simulink library "cooperative"  (Simulink 7.4)
settings: Solver=ode45  SolverMode=SingleTasking  StartTime=0.0  StopTime=10.0  RelTol=1e-3
undefined symbols (not defined in the file): ATRFunctions, g_AssignmentAlgorithm, g_CommandTurnRadius, g_CoordinationDelayDen, g_DefaultWaypointAltitude, g_EntityTypes, g_MaxNumberTargets, g_MaxNumberVehicles, g_MaxReassignmentDeltaTime, g_ObjectMessageIDs, g_OptionSaveDataAVDS, g_SampleTime, g_SensorRollLimitDeg, g_TargetStates, g_Tasks, g_TruthMemory, g_TypeAssignment, g_VehicleInputFiles, g_VehicleMemory, g_VehicleTypes, g_WaypointDefinitions, g_WaypointTypes
libraries: cooperative x23
(part 2 of 3)

== system cooperative/UAV1/SendMessages/SendATRTime ==
  VehicleID : Inport
  CommBusLocal : Inport  Port=2
  Bus Selector1 : BusSelector  OutputSignals=EFS(com).SensorManager(com).ATR Single.ATR Time
  CreateWaypointIndex : DataStoreMemory  DataStoreName=ATRTime
  Enabled Subsystem : Subsystem  TreatAsAtomicUnit=on
  Mux2 : Mux
  ReadWaypointIndex : DataStoreRead  DataStoreName=ATRTime  SampleTime=g_SampleTime
  Relational Operator : RelationalOperator  Operator=~=  InputSameDT=on
  SendATRTime : cooperative/SendMessage  ReuseMatrix=growing  MessageTypeStr=ATRTime
  Terminator : Terminator
  VehicleOffset : Constant  Value=g_ObjectMessageIDs.AllVehiclesTypeShifted + 1
  wires:
  Bus Selector1/1 -> Enabled Subsystem/1(ATRTime), Relational Operator/2, Mux2/3  "<ATR Time>"
  Enabled Subsystem/1(TimeStamp) -> Mux2/2  "TimeStamp"
  Mux2/1 -> SendATRTime/1
  Relational Operator/1 -> Enabled Subsystem/Enable
  ReadWaypointIndex/1 -> Relational Operator/1
  VehicleID/1 -> Mux2/1
  CommBusLocal/1 -> Bus Selector1/1
  VehicleOffset/1 -> Mux2/4
  SendATRTime/1 -> Terminator/1

== system cooperative/UAV1/SendMessages/SendAuctionData ==
  VehicleID : Inport
  CommBusLocal : Inport  Port=2
  Bus Selector1 : BusSelector  OutputSignals=EFS(com).CooperationManager(com).AuctionData.MessageNumber,EFS(com).CooperationManager(com).AuctionData.ReplanRound,EFS(com).CooperationManager(com).AuctionData.BidTarget,EFS(com).CooperationManager(com).AuctionData.BidPrice,EFS(com).CooperationManager(com).AuctionData.BidTargetETA,EFS(com).CooperationManager(com).AuctionData.AssignedTarget,EFS(com).CooperationManager(com).AuctionData.AssignedPrice,EFS(com).CooperationManager(com).AuctionData.AssignedTargetETA
  Data Store Memory : DataStoreMemory  DataStoreName=LastMessageNumber
  Data Store Read : DataStoreRead  DataStoreName=LastMessageNumber  SampleTime=g_SampleTime
  Enabled Subsystem : Subsystem  Priority=1  TreatAsAtomicUnit=on
  Mux2 : Mux  Inputs=11
  Relational Operator : RelationalOperator  Operator=~=  InputSameDT=on
  "SendAuctionData " : cooperative/SendMessage  Priority=2  ReuseMatrix=growing  MessageTypeStr=AuctionData
  Sum : Sum  Inputs=+  SaturateOnIntegerOverflow=on  InputSameDT=on  OutDataTypeStr=Inherit: Same as first input
  Terminator : Terminator
  VehicleOffset : Constant  Value=g_ObjectMessageIDs.AllVehiclesTypeShifted + 1
  wires:
  Bus Selector1/1 -> Enabled Subsystem/1(MessageNumber), Relational Operator/2  "<MessageNumber>"
  Bus Selector1/2 -> Mux2/4  "<ReplanRound>"
  Bus Selector1/3 -> Mux2/5  "<BidTarget>"
  Bus Selector1/4 -> Mux2/6  "<BidPrice>"
  Bus Selector1/5 -> Mux2/7  "<BidTargetETA>"
  Bus Selector1/6 -> Mux2/8  "<AssignedTarget>"
  Bus Selector1/7 -> Mux2/9  "<AssignedPrice>"
  Bus Selector1/8 -> Mux2/10  "<AssignedTargetETA>"
  Sum/1 -> Enabled Subsystem/Enable
  Relational Operator/1 -> Sum/1
  Data Store Read/1 -> Relational Operator/1
  Enabled Subsystem/1(TimeStamp) -> Mux2/3, Mux2/2  "TimeStamp"
  Mux2/1 -> "SendAuctionData "/1
  VehicleID/1 -> Mux2/1
  CommBusLocal/1 -> Bus Selector1/1
  VehicleOffset/1 -> Mux2/11
  "SendAuctionData "/1 -> Terminator/1

== system cooperative/UAV1/SendMessages/SendChangedStatus ==
  VehicleID : Inport
  CommBusLocal : Inport  Port=2
  Bus Selector1 : BusSelector  OutputSignals=EFS(com).TargetManager(com).Target Status.ChangedStatus
  Enabled Subsystem : Subsystem  TreatAsAtomicUnit=on
  Mux2 : Mux
  "SendChangedStatus " : cooperative/SendMessage  ReuseMatrix=growing  MessageTypeStr=ChangedStatus
  Terminator : Terminator
  VehicleOffset : Constant  Value=g_ObjectMessageIDs.AllVehiclesTypeShifted + 1
  wires:
  Bus Selector1/1 -> Enabled Subsystem/Enable, Mux2/3  "<ChangedStatus>"
  Enabled Subsystem/1(TimeStamp) -> Mux2/2  "TimeStamp"
  Mux2/1 -> "SendChangedStatus "/1
  VehicleID/1 -> Mux2/1
  CommBusLocal/1 -> Bus Selector1/1
  VehicleOffset/1 -> Mux2/4
  "SendChangedStatus "/1 -> Terminator/1

== system cooperative/UAV1/SendMessages/SendETAsCostsReturnToSearch ==
  VehicleID : Inport
  CommBusLocal : Inport  Port=2
  Bus Selector2 : BusSelector  OutputSignals=EFS(com).RouteManager(com).Replan ETAs and Costs.ReplanTime,EFS(com).RouteManager(com).Replan ETAs and Costs  OutputAsBus=on
  Mux : Mux  Inputs=3
  SendETAsCostsReturnToSearch : cooperative/SendMessage  ReuseMatrix=growing  MessageTypeStr=ETACostToSearch
  Terminator : Terminator
  VehicleOffset : Constant  Value=g_ObjectMessageIDs.AllVehiclesTypeShifted + 1
  wires:
  CommBusLocal/1 -> Bus Selector2/1
  VehicleID/1 -> Mux/1
  Mux/1 -> SendETAsCostsReturnToSearch/1
  Bus Selector2/1 -> Mux/2
  VehicleOffset/1 -> Mux/3
  SendETAsCostsReturnToSearch/1 -> Terminator/1

== system cooperative/UAV1/SendMessages/SendPositionFlag ==
  VehicleID : Inport
  CommBusLocal : Inport  Port=2
  CommBus : Inport  Port=3
  Bus Selector1 : BusSelector  OutputSignals=EFS(com).TargetManager(com).Target Status.NewTarget,EFS(com).RouteManager(com).NewPlans  OutputAsBus=on
  Bus Selector2 : BusSelector  OutputSignals=TimeTriggerReplan  OutputAsBus=on
  CreateWaypointIndex : DataStoreMemory  DataStoreName=PositionFlag  InitialValue=[0 0 0]
  Enabled Subsystem : Subsystem  TreatAsAtomicUnit=on
  Logical Operator1 : Logic  Operator=OR  Inputs=1
  Mux : Mux  Inputs=2
  Mux2 : Mux
  ReadWaypointIndex : DataStoreRead  DataStoreName=PositionFlag  SampleTime=g_SampleTime
  Relational Operator : RelationalOperator  Operator=~=  InputSameDT=on
  SendATRTime : cooperative/SendMessage  ReuseMatrix=growing  MessageTypeStr=SendPositionsFlag
  Terminator : Terminator
  VehicleOffset : Constant  Value=g_ObjectMessageIDs.AllVehiclesTypeShifted + 1
  wires:
  Mux/1 -> Enabled Subsystem/1(PositionFlag), Relational Operator/2
  Bus Selector1/1 -> Mux/1
  Bus Selector2/1 -> Mux/2
  CommBus/1 -> Bus Selector2/1
  Logical Operator1/1 -> Mux2/3, Enabled Subsystem/Enable
  Relational Operator/1 -> Logical Operator1/1
  CommBusLocal/1 -> Bus Selector1/1
  VehicleID/1 -> Mux2/1
  ReadWaypointIndex/1 -> Relational Operator/1
  Mux2/1 -> SendATRTime/1
  Enabled Subsystem/1(TimeStamp) -> Mux2/2  "TimeStamp"
  VehicleOffset/1 -> Mux2/4
  SendATRTime/1 -> Terminator/1

== system cooperative/UAV1/SendMessages/SendPositionID ==
  note: NOTE: Since the received messages are not reset to zero after they are handled, it was necessary to reset the PositionsFlag signal here.
      | The issue of resetting the message values to zero may be moved into the S-Function.
  VehicleID : Inport
  CommBusLocal : Inport  Port=2
  CommBus : Inport  Port=3
  Bus Selector1 : BusSelector  OutputSignals=Dynamics(com).AC Dynamics.Position_x,Dynamics(com).AC Dynamics.Position_y,Dynamics(com).AC Dynamics.Psi  OutputAsBus=on
  Bus Selector2 : BusSelector  OutputSignals=TimePositionsFlag  OutputAsBus=on
  Data Store Memory : DataStoreMemory  DataStoreName=PositionsSendFlagTime
  Data Store Read : DataStoreRead  DataStoreName=PositionsSendFlagTime  SampleTime=g_SampleTime
  Enabled Subsystem : Subsystem  TreatAsAtomicUnit=on
  Mux2 : Mux  Inputs=5
  Relational Operator : RelationalOperator  Operator=~=  InputSameDT=on
  "SendPositionID " : cooperative/SendMessage  ReuseMatrix=growing  MessageTypeStr=PositionID
  Terminator : Terminator
  VehicleOffset : Constant  Value=g_ObjectMessageIDs.AllVehiclesTypeShifted + 1
  wires:
  Relational Operator/1 -> Enabled Subsystem/Enable
  Data Store Read/1 -> Relational Operator/1
  Bus Selector2/1 -> Relational Operator/2, Enabled Subsystem/1(PositionSendFlag Time)
  CommBus/1 -> Bus Selector2/1
  CommBusLocal/1 -> Bus Selector1/1
  VehicleID/1 -> Mux2/3, Mux2/1
  Mux2/1 -> "SendPositionID "/1
  Enabled Subsystem/1(TimeStamp) -> Mux2/2  "TimeStamp"
  Bus Selector1/1 -> Mux2/4
  VehicleOffset/1 -> Mux2/5
  "SendPositionID "/1 -> Terminator/1

== system cooperative/UAV1/SendMessages/SendTargetAttacked ==
  VehicleID : Inport
  CommBusLocal : Inport  Port=2
  Bus Selector1 : BusSelector  OutputSignals=EFS(com).RouteManager(com).TaskStatus.Target Attacked
  CreateWaypointIndex : DataStoreMemory  DataStoreName=TargetAttacked
  Enabled Subsystem : Subsystem  TreatAsAtomicUnit=on
  Mux2 : Mux
  ReadWaypointIndex : DataStoreRead  DataStoreName=TargetAttacked  SampleTime=g_SampleTime
  Relational Operator : RelationalOperator  Operator=~=  InputSameDT=on
  "SendTargetAttacked " : cooperative/SendMessage  ReuseMatrix=growing  MessageTypeStr=TargetAttacked
  Terminator : Terminator
  VehicleOffset : Constant  Value=g_ObjectMessageIDs.AllVehiclesTypeShifted + 1
  wires:
  CommBusLocal/1 -> Bus Selector1/1
  VehicleID/1 -> Mux2/1
  ReadWaypointIndex/1 -> Relational Operator/1
  Relational Operator/1 -> Enabled Subsystem/Enable
  Mux2/1 -> "SendTargetAttacked "/1
  Enabled Subsystem/1(TimeStamp) -> Mux2/2  "TimeStamp"
  Bus Selector1/1 -> Mux2/3, Relational Operator/2, Enabled Subsystem/1("TargetAttacked ")  "<Target Attacked>"
  VehicleOffset/1 -> Mux2/4
  "SendTargetAttacked "/1 -> Terminator/1

== system cooperative/UAV1/SendMessages/SendTargetStatus ==
  VehicleID : Inport
  CommBusLocal : Inport  Port=2
  Bus Selector1 : BusSelector  OutputSignals=EFS(com).TargetManager(com).TargetStatusNoDelay.TargetStatus
  Bus Selector2 : BusSelector  OutputSignals=EFS(com).TargetManager(com).TargetStatusNoDelay.ChangedStatus
  Enabled Subsystem : Subsystem  Priority=1  TreatAsAtomicUnit=on
  Mux2 : Mux
  "SendTargetStatus " : cooperative/SendMessage  Priority=2  ReuseMatrix=growing  MessageTypeStr=TargetStatus
  Terminator : Terminator
  VehicleOffset : Constant  Value=g_ObjectMessageIDs.AllVehiclesTypeShifted + 1
  wires:
  Bus Selector2/1 -> Enabled Subsystem/Enable  "<ChangedStatus>"
  Bus Selector1/1 -> Mux2/3  "<TargetStatus>"
  Enabled Subsystem/1(TimeStamp) -> Mux2/2  "TimeStamp"
  Mux2/1 -> "SendTargetStatus "/1
  VehicleID/1 -> Mux2/1
  CommBusLocal/1 -> Bus Selector2/1, Bus Selector1/1
  VehicleOffset/1 -> Mux2/4
  "SendTargetStatus "/1 -> Terminator/1

== system cooperative/UAV1/SendMessages/SendTaskBenefits ==
  VehicleID : Inport
  CommBusLocal : Inport  Port=2
  Bus Selector1 : BusSelector  OutputSignals=EFS(com).CooperationManager(com).Algorithm Data.ReplanRound,EFS(com).CooperationManager(com).Algorithm Data.TargetStates,EFS(com).CooperationManager(com).Algorithm Data.TaskBenefits,EFS(com).CooperationManager(com).Algorithm Data.TimeToComplete,EFS(com).CooperationManager(com).Algorithm Data.SearchBenefit
  Data Store Memory : DataStoreMemory  DataStoreName=LastReplanRound  InitialValue=[0;0]
  Data Store Read : DataStoreRead  DataStoreName=LastReplanRound  SampleTime=g_SampleTime
  Enabled Subsystem : Subsystem  Priority=1  TreatAsAtomicUnit=on
  Mux2 : Mux  Inputs=8
  Relational Operator : RelationalOperator  Operator=~=  InputSameDT=on
  "SendTaskBenefits " : cooperative/SendMessage  Priority=2  ReuseMatrix=growing  MessageTypeStr=TaskBenefits
  Sum : Sum  Inputs=+  SaturateOnIntegerOverflow=on  InputSameDT=on  OutDataTypeStr=Inherit: Same as first input
  Terminator : Terminator
  VehicleOffset : Constant  Value=g_ObjectMessageIDs.AllVehiclesTypeShifted + 1
  wires:
  Bus Selector1/5 -> Mux2/7  "<SearchBenefit>"
  Bus Selector1/4 -> Mux2/6  "<TimeToComplete>"
  Bus Selector1/3 -> Mux2/5  "<TaskBenefits>"
  Sum/1 -> Enabled Subsystem/Enable
  Relational Operator/1 -> Sum/1
  Data Store Read/1 -> Relational Operator/1
  Bus Selector1/2 -> Mux2/4  "<TargetStates>"
  Bus Selector1/1 -> Enabled Subsystem/1(ReplanRound), Relational Operator/2, Mux2/3  "<ReplanRound>"
  Enabled Subsystem/1(TimeStamp) -> Mux2/2  "TimeStamp"
  Mux2/1 -> "SendTaskBenefits "/1
  VehicleID/1 -> Mux2/1
  CommBusLocal/1 -> Bus Selector1/1
  VehicleOffset/1 -> Mux2/8
  "SendTaskBenefits "/1 -> Terminator/1

== system cooperative/UAV1/SendMessages/SendTriggerReplan ==
  VehicleID : Inport
  CommBusLocal : Inport  Port=2
  Bus Selector1 : BusSelector  OutputSignals=EFS(com).RouteManager(com).TaskStatus.TriggerReplan  OutputAsBus=on
  Enabled Subsystem : Subsystem  TreatAsAtomicUnit=on
  Mux1 : Mux
  SendTriggerReplan : cooperative/SendMessage  ReuseMatrix=growing  MessageTypeStr=TriggerReplan
  Terminator : Terminator
  VehicleOffset : Constant  Value=g_ObjectMessageIDs.AllVehiclesTypeShifted + 1
  wires:
  Enabled Subsystem/1(TimeStamp) -> Mux1/2  "TriggerReplanTriggered"
  Bus Selector1/1 -> Enabled Subsystem/Enable, Mux1/3
  CommBusLocal/1 -> Bus Selector1/1
  VehicleID/1 -> Mux1/1
  Mux1/1 -> SendTriggerReplan/1
  VehicleOffset/1 -> Mux1/4
  SendTriggerReplan/1 -> Terminator/1

== system cooperative/UAV1/SendMessages/SendWaypointNumber ==
  VehicleID : Inport
  CommBusLocal : Inport  Port=2
  Bus Selector1 : BusSelector  OutputSignals=Dynamics(com).TacticalManuevering.WayPointNumber
  CreateWaypointIndex : DataStoreMemory  DataStoreName=WaypoinNumber  InitialValue=1
  Enabled Subsystem : Subsystem  TreatAsAtomicUnit=on
  Mux2 : Mux
  ReadWaypointIndex : DataStoreRead  DataStoreName=WaypoinNumber  SampleTime=g_SampleTime
  Relational Operator : RelationalOperator  Operator=~=  InputSameDT=on
  SendWaypointIndex : cooperative/SendMessage  ReuseMatrix=growing  MessageTypeStr=WaypointIndex
  Terminator : Terminator
  VehicleOffset : Constant  Value=g_ObjectMessageIDs.AllVehiclesTypeShifted + 1
  wires:
  CommBusLocal/1 -> Bus Selector1/1
  VehicleID/1 -> Mux2/1
  ReadWaypointIndex/1 -> Relational Operator/1
  Relational Operator/1 -> Enabled Subsystem/Enable
  Mux2/1 -> SendWaypointIndex/1
  Enabled Subsystem/1(TimeStamp) -> Mux2/2  "TimeStamp"
  Bus Selector1/1 -> Mux2/3, Relational Operator/2, Enabled Subsystem/1(Waypoint)  "<WayPointNumber>"
  VehicleOffset/1 -> Mux2/4
  SendWaypointIndex/1 -> Terminator/1

== system cooperative/UAV1/SendTruth/SendNewAssignment ==
  VehicleID : Inport
  SimmBusLocal : Inport  Port=2
  Bus Selector1 : BusSelector  OutputSignals=EFS(sim).CooperationManager(com).NewAssignmentTime
  Changed1 : Subsystem
  Enabled Subsystem : Subsystem  TreatAsAtomicUnit=on
  Mux2 : Mux
  Recipients : Constant  Value=[g_ObjectMessageIDs.AllVehiclesTypeShifted + 1]
  "SendTruth " : cooperative/SendTruth   ReuseMatrix=growing  MessageTypeStr=ChangeAssignmentFlagSelf
  Terminator : Terminator
  wires:
  "SendTruth "/1 -> Terminator/1
  Bus Selector1/1 -> Mux2/3, Changed1/1(Signal)  "<NewAssignmentTime>"
  Enabled Subsystem/1(TimeStamp) -> Mux2/2  "TimeStamp"
  Mux2/1 -> "SendTruth "/1
  VehicleID/1 -> Mux2/1
  Recipients/1 -> Mux2/4
  SimmBusLocal/1 -> Bus Selector1/1
  Changed1/1(Greater?) -> Enabled Subsystem/Enable

== system cooperative/UAV1/SendTruth/SendTargetStatus ==
  VehicleID : Inport
  CommBusLocal : Inport  Port=2
  Bus Selector2 : BusSelector  OutputSignals=EFS(com).TargetManager(com).Target Status.TargetStatus
  Data Store Memory : DataStoreMemory  DataStoreName=TargetStatus  InitialValue=zeros(g_MaxNumberTargets,1)
  Data Store Read : DataStoreRead  DataStoreName=TargetStatus  SampleTime=g_SampleTime
  Enabled Subsystem : Subsystem  TreatAsAtomicUnit=on
  Mux2 : Mux
  Recipients : Constant  Value=g_ObjectMessageIDs.DataSaveID + g_ObjectMessageIDs.MiscTypeShifted
  Relational Operator : RelationalOperator  Operator=~=  InputSameDT=on
  "SendTruth " : cooperative/SendTruth   ReuseMatrix=static  MessageTypeStr=TargetStatus
  Terminator : Terminator
  wires:
  Data Store Read/1 -> Relational Operator/1
  Relational Operator/1 -> Enabled Subsystem/Enable
  Enabled Subsystem/1(TimeStamp) -> Mux2/2  "TimeStamp"
  Mux2/1 -> "SendTruth "/1
  VehicleID/1 -> Mux2/1
  Recipients/1 -> Mux2/4
  CommBusLocal/1 -> Bus Selector2/1
  Bus Selector2/1 -> Mux2/3, Relational Operator/2, Enabled Subsystem/1(TargetStatus)  "<TargetStatus>"
  "SendTruth "/1 -> Terminator/1

== system cooperative/UAV1/SendTruth/SendTrackList ==
  VehicleID : Inport
  CommBusLocal : Inport  Port=2
  Bus Selector1 : BusSelector  OutputSignals=Dynamics(com).SensedTargets.SensedTargets,EFS(com).TargetManager(com).SensedTargetInformation.Targets  OutputAsBus=on
  Data Store Memory : DataStoreMemory  DataStoreName=TrackList  InitialValue=zeros(7*g_MaxNumberTargets,1)
  Data Store Read : DataStoreRead  DataStoreName=TrackList  SampleTime=g_SampleTime
  Enabled Subsystem : Subsystem  TreatAsAtomicUnit=on
  Mux : Mux  Inputs=2
  Mux2 : Mux  Inputs=5
  ObjectMode_temp : Constant
  ObjectType_temp : Constant
  Recipients : Constant  Value=g_ObjectMessageIDs.AllVehiclesTypeShifted + 1
  Relational Operator : RelationalOperator  Operator=~=  InputSameDT=on
  "SendTruth " : cooperative/SendTruth   ReuseMatrix=static  MessageTypeStr=TrackList
  Terminator : Terminator
  wires:
  Bus Selector1/1 -> Mux2/3, Enabled Subsystem/1(TrackList), Relational Operator/2
  Mux2/1 -> "SendTruth "/1
  VehicleID/1 -> Mux2/1
  CommBusLocal/1 -> Bus Selector1/1
  Recipients/1 -> Mux2/5
  Data Store Read/1 -> Relational Operator/1
  Relational Operator/1 -> Enabled Subsystem/Enable
  Enabled Subsystem/1(TimeStamp) -> Mux2/2
  "SendTruth "/1 -> Terminator/1
  Mux/1 -> Mux2/4
  ObjectMode_temp/1 -> Mux/2
  ObjectType_temp/1 -> Mux/1

== system cooperative/UAV1/SendTruth/SendTrueVehicleState ==
  VehicleID : Inport
  CommBusLocal : Inport  Port=2
  SimmBusLocal : Inport  Port=3
  Bus Selector1 : BusSelector  OutputSignals=Dynamics(com).AC Dynamics.Position_x,Dynamics(com).AC Dynamics.Position_y,Dynamics(com).AC Dynamics.Altitude,Dynamics(com).AC Dynamics.Phi,Dynamics(com).AC Dynamics.Theta,Dynamics(com).AC Dynamics.Psi  OutputAsBus=on
  Bus Selector2 : BusSelector  OutputSignals=EFS(sim).RouteManager(sim).VehicleFinished.Vehicle FinishedNoDelay  OutputAsBus=on
  Digital Clock : DigitalClock  SampleTime=g_SampleTime
  Mux2 : Mux  Inputs=5
  Recipients : Constant  Value=[g_ObjectMessageIDs.AllTargetsTypeShifted + 1,g_ObjectMessageIDs.DataSaveID + g_ObjectMessageIDs.MiscTypeShifted]
  "SendTruth " : cooperative/SendTruth   ReuseMatrix=static  MessageTypeStr=VehicleState
  Terminator : Terminator
  wires:
  Bus Selector1/1 -> Mux2/3
  Digital Clock/1 -> Mux2/2  "TimeStamp"
  Mux2/1 -> "SendTruth "/1
  VehicleID/1 -> Mux2/1
  CommBusLocal/1 -> Bus Selector1/1
  Recipients/1 -> Mux2/5
  "SendTruth "/1 -> Terminator/1
  SimmBusLocal/1 -> Bus Selector2/1
  Bus Selector2/1 -> Mux2/4

== system cooperative/UAV1/SendTruth/SendVehicleIsDead ==
  VehicleID : Inport
  SimmBusLocal : Inport  Port=2
  Bus Selector2 : BusSelector  OutputSignals=EFS(sim).RouteManager(sim).VehicleFinished.Vehicle FinishedNoDelay  OutputAsBus=on
  Create : DataStoreMemory  DataStoreName=VehicleIDead
  Enabled Subsystem : Subsystem  TreatAsAtomicUnit=on
  Mux2 : Mux  Inputs=3
  Read : DataStoreRead  DataStoreName=VehicleIDead  SampleTime=g_SampleTime
  Relational Operator : RelationalOperator  Operator=~=  InputSameDT=on
  "SendTruth " : cooperative/SendTruth   ReuseMatrix=static  MessageTypeStr=VehicleIsDead
  Terminator : Terminator
  wires:
  Bus Selector2/1 -> Mux2/3, Relational Operator/2, Enabled Subsystem/1(State)
  SimmBusLocal/1 -> Bus Selector2/1
  VehicleID/1 -> Mux2/1
  Mux2/1 -> "SendTruth "/1
  Relational Operator/1 -> Enabled Subsystem/Enable
  Read/1 -> Relational Operator/1
  Enabled Subsystem/1(TimeStamp) -> Mux2/2
  "SendTruth "/1 -> Terminator/1

== system cooperative/UAV1/SendTruth/SendWeaponsRelease ==
  VehicleID : Inport
  SimmBusLocal : Inport  Port=2
  Bus Selector1 : BusSelector  OutputSignals=EFS(sim).WeaponsManager(sim).BombDrop.BombID
  Bus Selector2 : BusSelector  OutputSignals=EFS(sim).WeaponsManager(sim).BombDrop
  Data Store Memory : DataStoreMemory  DataStoreName=WeaponID
  Data Store Read : DataStoreRead  DataStoreName=WeaponID  SampleTime=g_SampleTime
  Enabled Subsystem : Subsystem  TreatAsAtomicUnit=on
  Mux2 : Mux
  Recipients : Constant  Value=[g_ObjectMessageIDs.AllTargetsTypeShifted + 1]
  Relational Operator : RelationalOperator  Operator=~=  InputSameDT=on
  "SendTruth " : cooperative/SendTruth   ReuseMatrix=static  MessageTypeStr=WeaponsRelease
  Terminator : Terminator
  wires:
  SimmBusLocal/1 -> Bus Selector1/1, Bus Selector2/1
  Recipients/1 -> Mux2/4
  VehicleID/1 -> Mux2/1
  Mux2/1 -> "SendTruth "/1
  Enabled Subsystem/1(TimeStamp) -> Mux2/2  "TimeStamp"
  Relational Operator/1 -> Enabled Subsystem/Enable
  Data Store Read/1 -> Relational Operator/1
  Bus Selector1/1 -> Relational Operator/2, Enabled Subsystem/1(WeaponID)  "<BombID>"
  Bus Selector2/1 -> Mux2/3  "<BombDrop>"
  "SendTruth "/1 -> Terminator/1

== system cooperative/UAV1/SendTruth/VehicleStateSaveData ==
  VehicleID : Inport
  CommBusLocal : Inport  Port=2
  SimmBusLocal : Inport  Port=3
  Bus Selector1 : BusSelector  OutputSignals=Dynamics(com).AC Dynamics.Position_x,Dynamics(com).AC Dynamics.Position_y,Dynamics(com).AC Dynamics.Altitude,Dynamics(com).AC Dynamics.Phi,Dynamics(com).AC Dynamics.Theta,Dynamics(com).AC Dynamics.Psi,Dynamics(com).AC Dynamics.SensorOn,Dynamics(com).TacticalManuevering.RabbitNpos,Dynamics(com).TacticalManuevering.RabbitEpos,Dynamics(com).TacticalManuevering.RabbitHdg,Dynamics(com).TacticalManuevering.AssignedTarget  OutputAsBus=on
  Bus Selector2 : BusSelector  OutputSignals=EFS(sim).RouteManager(sim).VehicleFinished.Vehicle FinishedNoDelay  OutputAsBus=on
  Digital Clock : DigitalClock  SampleTime=g_SampleTime
  Mux2 : Mux  Inputs=5
  Recipients : Constant  Value=g_ObjectMessageIDs.DataSaveID + g_ObjectMessageIDs.MiscTypeShifted
  "SendTruth " : cooperative/SendTruth   ReuseMatrix=static  MessageTypeStr=VehicleStateSaveData
  Terminator : Terminator
  wires:
  Bus Selector2/1 -> Mux2/4
  SimmBusLocal/1 -> Bus Selector2/1
  Recipients/1 -> Mux2/5
  CommBusLocal/1 -> Bus Selector1/1
  VehicleID/1 -> Mux2/1
  Mux2/1 -> "SendTruth "/1
  Digital Clock/1 -> Mux2/2  "TimeStamp"
  Bus Selector1/1 -> Mux2/3
  "SendTruth "/1 -> Terminator/1

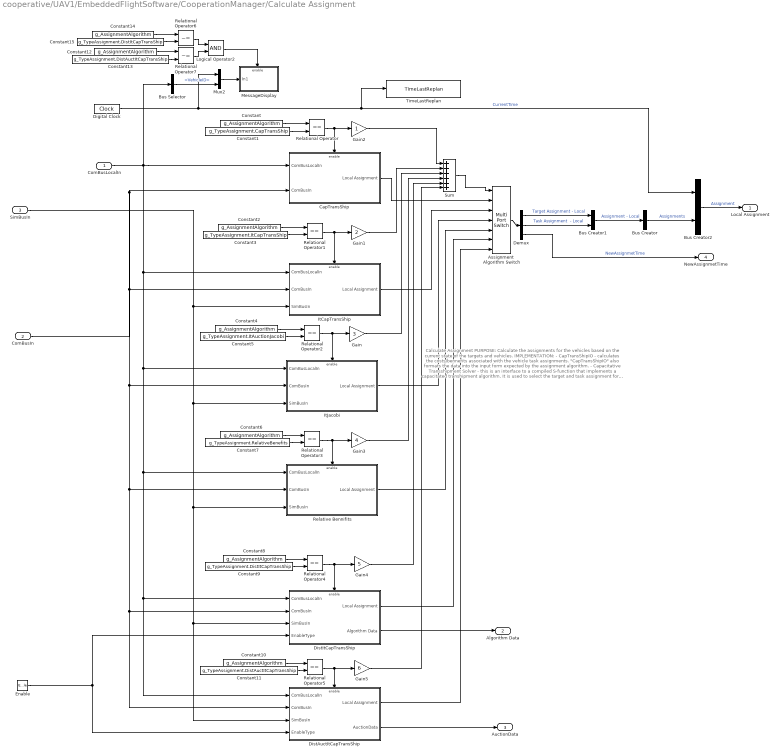
== system cooperative/UAV1/EmbeddedFlightSoftware/CooperationManager/Calculate Assignment ==
  note: Calculate Assignment
      |
      | PURPOSE: Calculate the assignments for the vehicles based on the current
      |      state of the targets and vehicles.
      |
      | IMPLEMENTATION:
      | - CapTransShipIO - calculates the costs/bennefits associated with the vehicle
      |      task assignments. "CapTransShipIO" also formats the data into the input
      |      form expected by the assignment algorithm.
      | - Capacitative Transshipment Solver - this is an interface to a compiled S-function
      |      that implements a capacitated transhipment algorithm. It is used to select the
      |      target and task assignment for all of the vehicles.
      | - Assignment for Local Vehicle - uses the current vehicle's ID to select and output
      |      the target and task assignment for this vehicle.
  ComBusLocalIn : Inport  SampleTime=g_SampleTime
  ComBusIn : Inport  Port=2  SampleTime=g_SampleTime
  SimBusIn : Inport  Port=3  SampleTime=g_SampleTime
  Enable : EnablePort  ShowOutputPort=on
  Assignment  Algorithm Switch : MultiPortSwitch  Inputs=6  SaturateOnIntegerOverflow=on  InputSameDT=on
  Bus Creator : BusCreator  Inputs=1
  Bus Creator1 : BusCreator  Inputs=2
  Bus Creator2 : BusCreator  Inputs=2
  Bus Selector : BusSelector  OutputSignals=VehicleID
  CapTransShip : Subsystem  TreatAsAtomicUnit=on
  Constant{,2,4,6,8,10,12,14} (8 alike) : Constant  Value=g_AssignmentAlgorithm
  Constant1 : Constant  Value=g_TypeAssignment.CapTransShip
  Constant11 : Constant  Value=g_TypeAssignment.DistAuctItCapTransShip
  Constant13 : Constant  Value=g_TypeAssignment.DistAuctItCapTransShip
  Constant15 : Constant  Value=g_TypeAssignment.DistItCapTransShip
  Constant3 : Constant  Value=g_TypeAssignment.ItCapTransShip
  Constant5 : Constant  Value=g_TypeAssignment.ItAuctionJacobi
  Constant7 : Constant  Value=g_TypeAssignment.RelativeBenefits
  Constant9 : Constant  Value=g_TypeAssignment.DistItCapTransShip
  Demux : Demux  Outputs=3
  Digital Clock : DigitalClock  SampleTime=g_SampleTime
  DistAuctItCapTransShip : Subsystem  TreatAsAtomicUnit=on
  DistItCapTransShip : Subsystem  TreatAsAtomicUnit=on
  Gain : Gain  Gain=3  SaturateOnIntegerOverflow=on  OutDataTypeStr=Inherit: Same as input  ParamDataTypeStr=Inherit: Same as input
  Gain1 : Gain  Gain=2  SaturateOnIntegerOverflow=on  OutDataTypeStr=Inherit: Same as input  ParamDataTypeStr=Inherit: Same as input
  Gain2 : Gain  SaturateOnIntegerOverflow=on  OutDataTypeStr=Inherit: Same as input  ParamDataTypeStr=Inherit: Same as input
  Gain3 : Gain  Gain=4  SaturateOnIntegerOverflow=on  OutDataTypeStr=Inherit: Same as input  ParamDataTypeStr=Inherit: Same as input
  Gain4 : Gain  Gain=5  SaturateOnIntegerOverflow=on  OutDataTypeStr=Inherit: Same as input  ParamDataTypeStr=Inherit: Same as input
  Gain5 : Gain  Gain=6  SaturateOnIntegerOverflow=on  OutDataTypeStr=Inherit: Same as input  ParamDataTypeStr=Inherit: Same as input
  ItCapTransShip : Subsystem  TreatAsAtomicUnit=on
  ItJacobi : Subsystem  TreatAsAtomicUnit=on
  Logical Operator2 : Logic
  MessageDisplay : Subsystem  TreatAsAtomicUnit=on
  Mux2 : Mux  Inputs=2
  Relational Operator{,1..5} (6 alike) : RelationalOperator  Operator===  InputSameDT=on
  Relational Operator6 : RelationalOperator  Operator=~=  InputSameDT=on
  Relational Operator7 : RelationalOperator  Operator=~=  InputSameDT=on
  Relative Bennifits : Subsystem  TreatAsAtomicUnit=on
  Sum : Sum  Inputs=++++++  SaturateOnIntegerOverflow=on  InputSameDT=on  OutDataTypeStr=Inherit: Same as first input
  TimeLastReplan : DataStoreWrite  DataStoreName=TimeLastReplan  SampleTime=g_SampleTime
  Local Assignment : Outport
  Algorithm Data : Outport  Port=2
  AuctionData : Outport  Port=3
  NewAssignmetTime : Outport  Port=4
  wires:
  Enable/1 -> DistAuctItCapTransShip/4(EnableType), DistItCapTransShip/4(EnableType)
  Logical Operator2/1 -> MessageDisplay/Enable
  Relational Operator7/1 -> Logical Operator2/2
  Relational Operator6/1 -> Logical Operator2/1
  Constant13/1 -> Relational Operator7/2
  Constant12/1 -> Relational Operator7/1
  Constant15/1 -> Relational Operator6/2
  Constant14/1 -> Relational Operator6/1
  DistAuctItCapTransShip/2(AuctionData) -> AuctionData/1
  Gain5/1 -> Sum/6
  DistAuctItCapTransShip/1(Local Assignment) -> Assignment  Algorithm Switch/7
  Constant11/1 -> Relational Operator5/2
  Constant10/1 -> Relational Operator5/1
  Relational Operator5/1 -> DistAuctItCapTransShip/Enable, Gain5/1
  DistItCapTransShip/2(Algorithm Data) -> Algorithm Data/1
  DistItCapTransShip/1(Local Assignment) -> Assignment  Algorithm Switch/6
  Gain4/1 -> Sum/5
  Constant9/1 -> Relational Operator4/2
  Constant8/1 -> Relational Operator4/1
  Relational Operator4/1 -> DistItCapTransShip/Enable, Gain4/1
  Bus Selector/1 -> Mux2/2  "<VehicleID>"
  Mux2/1 -> MessageDisplay/1(In1)
  SimBusIn/1 -> DistAuctItCapTransShip/3(SimBusIn), DistItCapTransShip/3(SimBusIn), Relative Bennifits/3(SimBusIn), ItJacobi/3(SimBusIn), ItCapTransShip/3(SimBusIn)
  Demux/2 -> Bus Creator1/2  "Task Assignment  - Local"
  Demux/1 -> Bus Creator1/1  "Target Assignment - Local"
  Bus Creator1/1 -> Bus Creator/1  "Assignment - Local"
  Assignment  Algorithm Switch/1 -> Demux/1
  Gain3/1 -> Sum/4
  Constant7/1 -> Relational Operator3/2
  Constant6/1 -> Relational Operator3/1
  Relational Operator3/1 -> Relative Bennifits/Enable, Gain3/1
  Relative Bennifits/1(Local Assignment) -> Assignment  Algorithm Switch/5
  Gain/1 -> Sum/3
  Gain1/1 -> Sum/2
  Gain2/1 -> Sum/1
  Sum/1 -> Assignment  Algorithm Switch/1
  Constant5/1 -> Relational Operator2/2
  Constant4/1 -> Relational Operator2/1
  Relational Operator2/1 -> ItJacobi/Enable, Gain/1
  ItJacobi/1(Local Assignment) -> Assignment  Algorithm Switch/4
  Constant3/1 -> Relational Operator1/2
  Constant2/1 -> Relational Operator1/1
  Relational Operator1/1 -> Gain1/1, ItCapTransShip/Enable
  ItCapTransShip/1(Local Assignment) -> Assignment  Algorithm Switch/3
  Constant1/1 -> Relational Operator/2
  Constant/1 -> Relational Operator/1
  Relational Operator/1 -> Gain2/1, CapTransShip/Enable
  ComBusLocalIn/1 -> Bus Selector/1, CapTransShip/1(ComBusLocalIn), DistItCapTransShip/1(ComBusLocalIn), DistAuctItCapTransShip/1(ComBusLocalIn), Relative Bennifits/1(ComBusLocalIn), ItJacobi/1(ComBusLocalIn), ItCapTransShip/1(ComBusLocalIn)
  CapTransShip/1(Local Assignment) -> Assignment  Algorithm Switch/2
  Bus Creator/1 -> Bus Creator2/2  "Assignments"
  ComBusIn/1 -> DistItCapTransShip/2(ComBusIn), DistAuctItCapTransShip/2(ComBusIn), Relative Bennifits/2(ComBusIn), ItJacobi/2(ComBusIn), ItCapTransShip/2(ComBusIn), CapTransShip/2(ComBusIn)
  Digital Clock/1 -> Mux2/1, TimeLastReplan/1, Bus Creator2/1  "CurrentTime"
  Bus Creator2/1 -> Local Assignment/1  "Assignment"
  Demux/3 -> NewAssignmetTime/1  "NewAssignmetTime"

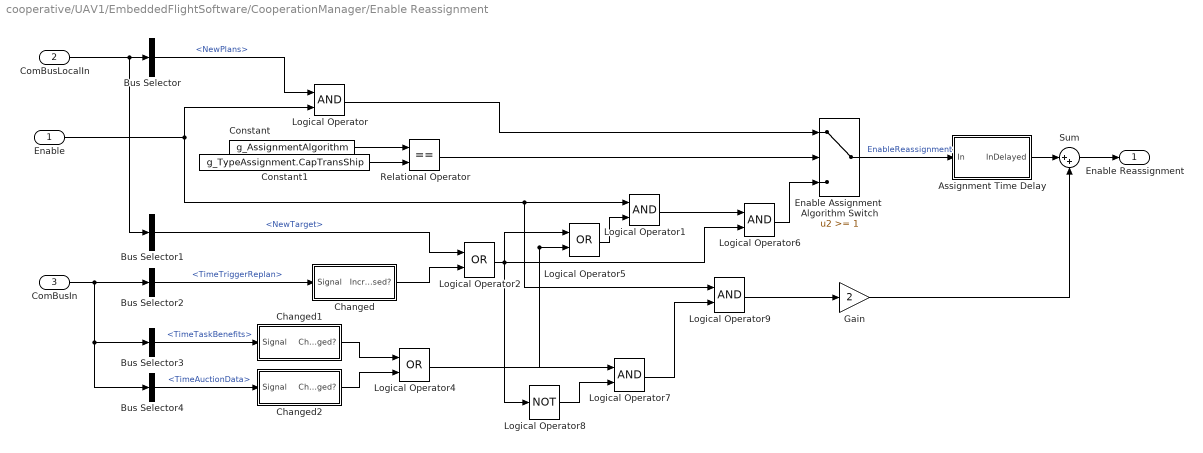
== system cooperative/UAV1/EmbeddedFlightSoftware/CooperationManager/Enable Reassignment ==
  Enable : Inport  SampleTime=g_SampleTime
  ComBusLocalIn : Inport  Port=2  SampleTime=g_SampleTime
  ComBusIn : Inport  Port=3  SampleTime=g_SampleTime
  Assignment Time Delay : Subsystem
  Bus Selector : BusSelector  OutputSignals=EFS(com).RouteManager(com).NewPlans
  Bus Selector1 : BusSelector  OutputSignals=EFS(com).TargetManager(com).Target Status.NewTarget
  Bus Selector2 : BusSelector  OutputSignals=TimeTriggerReplan
  Bus Selector3 : BusSelector  OutputSignals=TimeTaskBenefits
  Bus Selector4 : BusSelector  OutputSignals=TimeAuctionData
  Changed : Subsystem
  Changed1 : Subsystem
  Changed2 : Subsystem
  Constant : Constant  Value=g_AssignmentAlgorithm
  Constant1 : Constant  Value=g_TypeAssignment.CapTransShip
  Enable Assignment  Algorithm Switch : Switch  Threshold=1  SaturateOnIntegerOverflow=on  InputSameDT=on
  Gain : Gain  Gain=2  SaturateOnIntegerOverflow=on  OutDataTypeStr=Inherit: Same as input  ParamDataTypeStr=Inherit: Same as input
  Logical Operator{,1,6..7,9} (5 alike) : Logic
  Logical Operator2 : Logic  Operator=OR
  Logical Operator4 : Logic  Operator=OR
  Logical Operator5 : Logic  Operator=OR
  Logical Operator8 : Logic  Operator=NOT
  Relational Operator : RelationalOperator  Operator===  InputSameDT=on
  Sum : Sum  Inputs=|++  SaturateOnIntegerOverflow=on  InputSameDT=on  OutDataTypeStr=Inherit: Same as first input
  Enable Reassignment : Outport
  wires:
  Sum/1 -> Enable Reassignment/1
  Gain/1 -> Sum/2
  Assignment Time Delay/1(InDelayed) -> Sum/1
  Logical Operator9/1 -> Gain/1
  Logical Operator7/1 -> Logical Operator9/2
  Logical Operator8/1 -> Logical Operator7/2
  Logical Operator2/1 -> Logical Operator8/1, Logical Operator6/2, Logical Operator5/1
  Logical Operator5/1 -> Logical Operator1/2
  Logical Operator4/1 -> Logical Operator5/2, Logical Operator7/1
  Changed/1(Increased?) -> Logical Operator2/2
  ComBusIn/1 -> Bus Selector2/1, Bus Selector3/1, Bus Selector4/1
  Bus Selector1/1 -> Logical Operator2/1  "<NewTarget>"
  Logical Operator/1 -> Enable Assignment  Algorithm Switch/1
  Constant1/1 -> Relational Operator/2
  Constant/1 -> Relational Operator/1
  Relational Operator/1 -> Enable Assignment  Algorithm Switch/2
  Enable/1 -> Logical Operator/2, Logical Operator1/1, Logical Operator9/1
  ComBusLocalIn/1 -> Bus Selector1/1, Bus Selector/1
  Bus Selector/1 -> Logical Operator/1  "<NewPlans>"
  Logical Operator1/1 -> Logical Operator6/1
  Bus Selector2/1 -> Changed/1(Signal)  "<TimeTriggerReplan>"
  Logical Operator6/1 -> Enable Assignment  Algorithm Switch/3
  Enable Assignment  Algorithm Switch/1 -> Assignment Time Delay/1(In)  "EnableReassignment"
  Bus Selector3/1 -> Changed1/1(Signal)  "<TimeTaskBenefits>"
  Changed1/1(Changed?) -> Logical Operator4/1
  Bus Selector4/1 -> Changed2/1(Signal)  "<TimeAuctionData>"
  Changed2/1(Changed?) -> Logical Operator4/2

== system cooperative/UAV1/EmbeddedFlightSoftware/CooperationManager/Task List ==
  ComBusLocalIn : Inport
  Bus Selector : BusSelector  OutputSignals=EFS(com).TargetManager(com).Target Status.TargetStatus
  Bus Selector1 : BusSelector  OutputSignals=VehicleID
  Check for Changed  Target Status : RelationalOperator  Operator=~=  InputSameDT=on
  Constant : Constant  Value=0
  Create Last  Target Status : DataStoreMemory  DataStoreName=LastTargetStatus  InitialValue=[1:(g_MaxNumberTargets)]*-1
  Read Last  LastTargetStatus : DataStoreRead  DataStoreName=LastTargetStatus  SampleTime=g_SampleTime
  Switch : Switch  Threshold=0.5  SaturateOnIntegerOverflow=on  InputSameDT=on
  Update Task List : Subsystem  TreatAsAtomicUnit=on
  or 1 : Logic  Operator=OR  Inputs=1
  UnassignTaskFlag : Outport
  wires:
  Update Task List/1(UnassignedTaskFlag) -> Switch/1
  Constant/1 -> Switch/3
  Switch/1 -> UnassignTaskFlag/1
  ComBusLocalIn/1 -> Bus Selector1/1, Bus Selector/1
  Bus Selector1/1 -> Update Task List/1(Vehicle ID)  "<VehicleID>"
  or 1/1 -> Switch/2, Update Task List/Enable
  Bus Selector/1 -> Update Task List/2(TargetStatus), Check for Changed  Target Status/2  "<TargetStatus>"
  Check for Changed  Target Status/1 -> or 1/1  "ChangedTargetStatus"
  Read Last  LastTargetStatus/1 -> Check for Changed  Target Status/1  "LastTargetStatus"

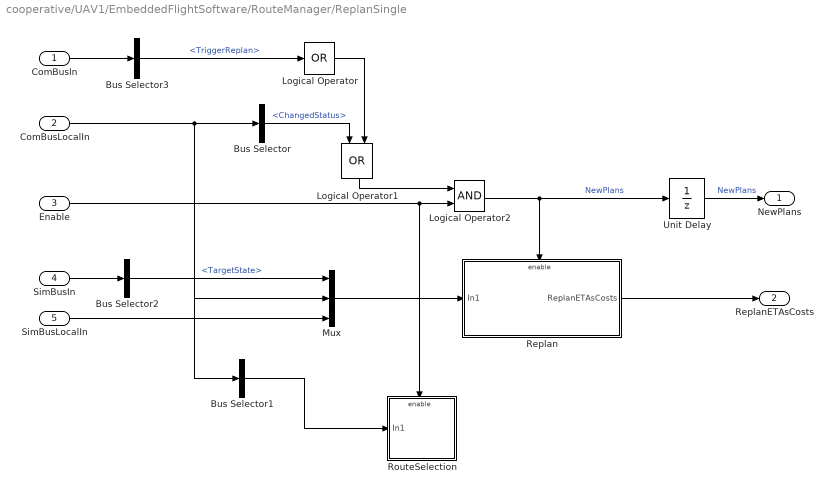
== system cooperative/UAV1/EmbeddedFlightSoftware/RouteManager/ReplanSingle ==
  ComBusIn : Inport
  ComBusLocalIn : Inport  Port=2
  Enable : Inport  Port=3
  SimBusIn : Inport  Port=4
  SimBusLocalIn : Inport  Port=5
  Bus Selector : BusSelector  OutputSignals=EFS(com).TargetManager(com).Target Status.ChangedStatus
  Bus Selector1 : BusSelector  OutputSignals="VehicleID,Time,EFS(com).CooperationManager(com).Assignment.Assignments.Assignment - Local.Target Assignment - Local,EFS(com).CooperationManager(com).Assignment.Assignments.Assignment - Local.Task Assignment  - Local,Dynamics(com).TacticalManuevering.WayPointNumber,EFS(com).RouteManager(com).TaskStatus.Task Finished,Dynamics(com).AC Dynamics.Position_x,Dynamics(com).AC Dynamics.Position_y,Dynamics(com).AC Dynamics.Altitude,Dynamics(com).AC Dynamics.Psi,Dynamics(com).AC Dynamics.V North,Dynamics(com).AC Dynamics.V East,Dynamics(com).TacticalManuevering.CommandTurnRadius,Dynamics(com).TacticalManuevering.CommandVelocity"  OutputAsBus=on
  Bus Selector2 : BusSelector  OutputSignals=ExternalTruth.TargetState
  Bus Selector3 : BusSelector  OutputSignals=TriggerReplan
  Logical Operator : Logic  Operator=OR  Inputs=1
  Logical Operator1 : Logic  Operator=OR
  Logical Operator2 : Logic
  Mux : Mux  Inputs=3
  Replan : Subsystem  TreatAsAtomicUnit=on
  RouteSelection : Subsystem  TreatAsAtomicUnit=on
  Unit Delay : UnitDelay  SampleTime=g_SampleTime
  NewPlans : Outport
  ReplanETAsCosts : Outport  Port=2
  wires:
  Bus Selector3/1 -> Logical Operator/1  "<TriggerReplan>"
  SimBusLocalIn/1 -> Mux/3
  Replan/1(ReplanETAsCosts) -> ReplanETAsCosts/1
  SimBusIn/1 -> Bus Selector2/1
  Unit Delay/1 -> NewPlans/1  "NewPlans"
  ComBusIn/1 -> Bus Selector3/1
  ComBusLocalIn/1 -> Bus Selector1/1, Mux/2, Bus Selector/1
  Logical Operator2/1 -> Replan/Enable, Unit Delay/1  "NewPlans"
  Enable/1 -> Logical Operator2/2, RouteSelection/Enable
  Bus Selector1/1 -> RouteSelection/1(In1)
  Logical Operator1/1 -> Logical Operator2/1
  Logical Operator/1 -> Logical Operator1/2
  Bus Selector/1 -> Logical Operator1/1  "<ChangedStatus>"
  Bus Selector2/1 -> Mux/1  "<TargetState>"
  Mux/1 -> Replan/1(In1)

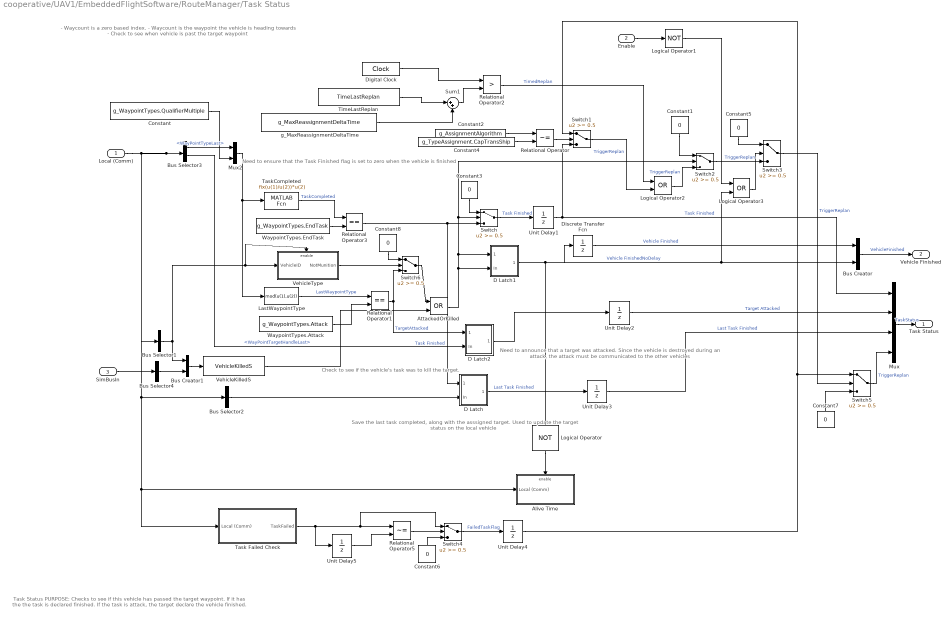
== system cooperative/UAV1/EmbeddedFlightSoftware/RouteManager/Task Status ==
  note: - Waycount is a zero based index.
      | - Waycount is the waypoint the vehicle is
      | heading towards
      | - Check to see when vehicle is past the
      | target waypoint
  note: Need to ensure that the Task Finished
      | flag is set to zero when the vehicle is finished
  note: Check to see if the vehicle's
      | task was to kill the target.
  note: Need to announce that a target was
      | attacked. Since the vehicle is destroyed
      | during an attack, the attack must be
      | communicated to the other vehicles
  note: Save the last task completed,
      | along with the asssigned target.
      | Used to update the target status
      | on the local vehicle
  note: Task Status
      |
      | PURPOSE: Checks to see if this vehicle has passed the target waypoint. If it
      | has the the task is declared finished. If the task is attack, the target declare the
      | vehicle finished.
  Local (Comm) : Inport  SampleTime=g_SampleTime
  Enable : Inport  Port=2  SampleTime=g_SampleTime
  SimBusIn : Inport  Port=3  SampleTime=g_SampleTime
  Alive Time : Subsystem  TreatAsAtomicUnit=on
  AttackedOrKilled : Logic  Operator=OR
  Bus Creator : BusCreator  Inputs=2
  Bus Creator1 : BusCreator  Inputs=2
  Bus Selector1 : BusSelector  OutputSignals=VehicleID  OutputAsBus=on
  Bus Selector2 : BusSelector  OutputSignals=Dynamics(com).TacticalManuevering.AssignedTarget,Dynamics(com).TacticalManuevering.AssignedTask  OutputAsBus=on
  Bus Selector3 : BusSelector  OutputSignals=Dynamics(com).TacticalManuevering.WayPointTypeLast,Dynamics(com).TacticalManuevering.WayPointTargetHandleLast
  Bus Selector4 : BusSelector  OutputSignals=ExternalTruth.VehicleKilled  OutputAsBus=on
  Constant : Constant  Value=g_WaypointTypes.QualifierMultiple
  Constant{1,3,5..8} (6 alike) : Constant  Value=0
  Constant2 : Constant  Value=g_AssignmentAlgorithm
  Constant4 : Constant  Value=g_TypeAssignment.CapTransShip
  D Latch : Subsystem
      mask Type: DLatch
      mask Description: D Latch Flip Flop Block
  D Latch1 : Subsystem
      mask Type: DLatch
      mask Description: D Latch Flip Flop Block
  D Latch2 : Subsystem
      mask Type: DLatch
      mask Description: D Latch Flip Flop Block
  Digital Clock : DigitalClock  SampleTime=g_SampleTime
  Discrete Transfer Fcn : DiscreteTransferFcn  Denominator=[1 0 ]  SampleTime=g_SampleTime
  LastWaypointType : MATLABFcn  MATLABFcn=mod(u(1),u(2))
  Logical Operator : Logic  Operator=NOT
  Logical Operator1 : Logic  Operator=NOT
  Logical Operator2 : Logic  Operator=OR
  Logical Operator3 : Logic  Operator=OR
  Mux : Mux  Inputs=[1 1 2 1]
  Mux2 : Mux  Inputs=2
  Relational Operator : RelationalOperator  Operator=~=  InputSameDT=on
  Relational Operator1 : RelationalOperator  Operator===  InputSameDT=on
  Relational Operator2 : RelationalOperator  Operator=>  InputSameDT=on
  Relational Operator3 : RelationalOperator  Operator===  InputSameDT=on
  Relational Operator5 : RelationalOperator  Operator=~=  InputSameDT=on
  Sum1 : Sum  Inputs=|++  SaturateOnIntegerOverflow=on  InputSameDT=on  OutDataTypeStr=Inherit: Same as first input
  Switch{,1..6} (7 alike) : Switch  Threshold=0.5  SaturateOnIntegerOverflow=on  InputSameDT=on
  Task Failed Check : Subsystem  TreatAsAtomicUnit=on
  TaskCompleted : MATLABFcn  MATLABFcn=fix(u(1)/u(2))*u(2)
  TimeLastReplan : DataStoreRead  DataStoreName=TimeLastReplan  SampleTime=g_SampleTime
  Unit Delay{1..5} (5 alike) : UnitDelay  SampleTime=g_SampleTime
  VehicleKilledS : S-Function  FunctionName=VehicleKilledS  Parameters=g_MaxNumberVehicles, g_MaxNumberTargets  EnableBusSupport=off
  VehicleType : Subsystem  TreatAsAtomicUnit=on
  WaypointTypes.Attack : Constant  Value=g_WaypointTypes.Attack
  WaypointTypes.EndTask : Constant  Value=g_WaypointTypes.EndTask
  g_MaxReassignmentDeltaTime : Constant  Value=g_MaxReassignmentDeltaTime
  Task Status : Outport
  Vehicle Finished : Outport  Port=2
  wires:
  Constant7/1 -> Switch5/3
  Switch5/1 -> Mux/4  "TriggerReplan"
  Unit Delay4/1 -> Switch5/1, Switch1/1
  Relational Operator2/1 -> Logical Operator2/1  "TimedReplan"
  Constant6/1 -> Switch4/3
  Switch4/1 -> Unit Delay4/1  "FailedTaskFlag"
  Unit Delay5/1 -> Relational Operator5/2
  Task Failed Check/1(TaskFailed) -> Switch4/1, Relational Operator5/1, Unit Delay5/1
  Local (Comm)/1 -> Task Failed Check/1(Local (Comm)), Alive Time/1(Local (Comm)), Bus Selector2/1, Bus Selector1/1, Bus Selector3/1
  WaypointTypes.EndTask/1 -> Relational Operator3/2
  WaypointTypes.Attack/1 -> Relational Operator1/2
  Constant3/1 -> Switch/1
  Switch/1 -> Unit Delay1/1  "Task Finished"
  Bus Selector2/1 -> D Latch/2(In)
  Relational Operator3/1 -> D Latch/1(Enable), Switch/3  "Task Finished"
  Mux/1 -> Task Status/1  "TaskStatus"
  D Latch/1(Latched) -> Unit Delay3/1  "Last Task Finished"
  Discrete Transfer Fcn/1 -> Bus Creator/1  "Vehicle Finished"
  Unit Delay1/1 -> Switch1/3, Mux/1  "Task Finished"
  Unit Delay2/1 -> Mux/2  "Target Attacked"
  D Latch1/1(Latched) -> Discrete Transfer Fcn/1, Logical Operator/1, Bus Creator/2, Logical Operator3/2  "Vehicle FinishedNoDelay"
  Unit Delay3/1 -> Mux/3  "Last Task Finished"
  Bus Creator/1 -> Vehicle Finished/1  "VehicleFinished"
  Constant1/1 -> Switch2/1
  Logical Operator2/1 -> Switch2/3  "TriggerReplan"
  Bus Selector3/1 -> Mux2/1  "<WayPointTypeLast>"
  LastWaypointType/1 -> Relational Operator1/1  "LastWaypointType"
  TaskCompleted/1 -> Relational Operator3/1  "TaskCompleted"
  Constant/1 -> Mux2/2
  Mux2/1 -> LastWaypointType/1, TaskCompleted/1
  Bus Selector3/2 -> D Latch2/2(In)  "<WayPointTargetHandleLast>"
  D Latch2/1(Latched) -> Unit Delay2/1
  Logical Operator/1 -> Alive Time/Enable
  Relational Operator/1 -> Switch1/2
  Constant2/1 -> Relational Operator/1
  Constant4/1 -> Relational Operator/2
  Switch1/1 -> Logical Operator2/2  "TriggerReplan"
  Switch2/1 -> Switch3/3  "TriggerReplan"
  Relational Operator5/1 -> Switch4/2
  Sum1/1 -> Relational Operator2/2
  g_MaxReassignmentDeltaTime/1 -> Sum1/2
  TimeLastReplan/1 -> Sum1/1
  Digital Clock/1 -> Relational Operator2/1
  Constant5/1 -> Switch3/1
  Switch3/1 -> Switch5/2  "TriggerReplan"
  Logical Operator1/1 -> Logical Operator3/1
  Enable/1 -> Logical Operator1/1
  Logical Operator3/1 -> Switch3/2
  Bus Selector1/1 -> Bus Creator1/1, VehicleType/1(VehicleID), VehicleType/Enable
  Relational Operator1/1 -> Switch6/3, D Latch2/1(Enable)  "TargetAttacked"
  VehicleKilledS/1 -> AttackedOrKilled/2
  AttackedOrKilled/1 -> D Latch1/2(In), D Latch1/1(Enable), Switch2/2, Switch/2
  Bus Creator1/1 -> VehicleKilledS/1
  Bus Selector4/1 -> Bus Creator1/2
  SimBusIn/1 -> Bus Selector4/1
  Constant8/1 -> Switch6/1
  VehicleType/1(NotMunition) -> Switch6/2
  Switch6/1 -> AttackedOrKilled/1

== system cooperative/UAV1/EmbeddedFlightSoftware/SensorManager/ATR Combined ==
  note: ATR Combined
      |
      | PURPOSE: Used to calculate a  combined ATR value for
      |      each target using single ATRs from this and other vehicles.
      |
      | IMPLEMENTATION:
      | - ATRCombined - calls the function "ATRFunctions" to calculate
      |      combined ATR values for the targets.
      | - Write ATR Memory - saves the last values of the single ATRs
      |       to enable a check for changes in these values.
  In1 : Inport  SampleTime=g_SampleTime
  In2 : Inport  Port=2  SampleTime=g_SampleTime
  Enable : EnablePort
  ATRCombined : S-Function  FunctionName=ATRFunctionsCombinedS  Parameters=g_MaxNumberTargets  EnableBusSupport=off
  Bus Creator : BusCreator
  Bus Creator1 : BusCreator
  Demux : Demux  Outputs=[g_MaxNumberTargets,g_MaxNumberTargets,g_MaxNumberTargets,g_MaxNumberTargets,g_MaxNumberTargets,g_MaxNumberTargets]
  Digital Clock : DigitalClock  SampleTime=g_SampleTime
  Write ATR Memory : DataStoreWrite  DataStoreName=ATRMemory  SampleTime=g_SampleTime
  Out1 : Outport
  wires:
  Demux/6 -> Bus Creator1/4  "NumberValidHeadings"
  Demux/5 -> Bus Creator/4  "DesiredHeadings04"
  Demux/4 -> Bus Creator/3  "DesiredHeadings03"
  Demux/3 -> Bus Creator/2  "DesiredHeadings02"
  Demux/2 -> Bus Creator/1  "DesiredHeadings01"
  In1/1 -> ATRCombined/1
  In2/1 -> Write ATR Memory/1
  Digital Clock/1 -> Bus Creator1/1  "ATR Combined Time"
  Bus Creator1/1 -> Out1/1  "ATR Combined"
  Demux/1 -> Bus Creator1/2  "CombinedATRValues"
  Bus Creator/1 -> Bus Creator1/3  "Desired Headings"
  ATRCombined/1 -> Demux/1  "ATR Combined"

== system cooperative/UAV1/EmbeddedFlightSoftware/SensorManager/ATR Single ==
  note: ATR Single
      |
      | PURPOSE: This block  is used to calculate a  value for ATR
      |      for a given target based on sensor data from this vehicle.
      |
      | IMPLEMENTATION:
      | - Automatic Target Recognition (ATR) - calls the M-function,
      |      "ATRFunctions" to calculation the single ATR value.
      | - Save Last Sensor Update - saves the last sensed values of the targets from
      |      the local vehicle to enable a check for changes in these values.
  VehicleID Psi SensedTargets : Inport  SampleTime=g_SampleTime
  Target Truth : Inport  Port=2  SampleTime=g_SampleTime
  SendFlag : Inport  Port=3  SampleTime=g_SampleTime
  TargetStatus : Inport  Port=4  SampleTime=g_SampleTime
  Enable : EnablePort
  Bus Selector : BusSelector  OutputSignals=SensedTargets
  Save Last Sensor Update : DataStoreWrite  DataStoreName=LastSensorUpdate  SampleTime=g_SampleTime
  SingleATR : Subsystem  TreatAsAtomicUnit=on
  ATR Single : Outport
  wires:
  TargetStatus/1 -> SingleATR/3(TargetStatus)
  SendFlag/1 -> SingleATR/Enable
  Bus Selector/1 -> Save Last Sensor Update/1  "<SensedTargets>"
  Target Truth/1 -> SingleATR/2("Target Truth ")
  SingleATR/1(Out1) -> ATR Single/1
  VehicleID Psi SensedTargets/1 -> SingleATR/1(VehicleID Psi), Bus Selector/1

== system cooperative/UAV1/EmbeddedFlightSoftware/SensorManager/BDA ==
  note: BDA
      |
      | PURPOSE: This block  is used to calculate a  value for BDA for a
      |      given target based on sensor data from this vehicle. The block "
      |
      | IMPLEMENTATION:
      | - BDA Calculation - calls the M-function, "ATRFunctions" to calculate
      |      a BDA value if it is appropriate to do so.
  VehicleID Psi SensedTargets : Inport  SampleTime=g_SampleTime
  Target Truth : Inport  Port=2  SampleTime=g_SampleTime
  Local (Comm) : Inport  Port=3  SampleTime=g_SampleTime
  SimBusIn : Inport  Port=4  SampleTime=g_SampleTime
  Enable : EnablePort
  BDA Calculation : MATLABFcn  MATLABFcn=ATRFunctions('BDA',u)  OutputDimensions=g_MaxNumberTargets
  Bus Selector : BusSelector  OutputSignals=SensedTargets
  Bus Selector1 : BusSelector  OutputSignals=VehicleID,EFS(com).TargetManager(com).Target Status.TargetStatus  OutputAsBus=on
  Bus Selector2 : BusSelector  OutputSignals=ExternalTruth.TargetState
  Mux2 : Mux
  BDA : Outport
  wires:
  VehicleID Psi SensedTargets/1 -> Bus Selector/1
  Target Truth/1 -> Mux2/3
  Bus Selector/1 -> Mux2/2  "<SensedTargets>"
  Mux2/1 -> BDA Calculation/1
  Local (Comm)/1 -> Bus Selector1/1
  Bus Selector1/1 -> Mux2/1
  SimBusIn/1 -> Bus Selector2/1
  Bus Selector2/1 -> Mux2/4  "<TargetState>"
  BDA Calculation/1 -> BDA/1  "BDA"

== system cooperative/UAV1/EmbeddedFlightSoftware/TargetManager/New Target Check ==
  TargetStatus : Inport
  And 1 : Logic
  And 3 : Logic  Operator=OR  Inputs=1
  Check for new target : RelationalOperator  Operator===  InputSameDT=on
  Check for new target1 : RelationalOperator  Operator=~=  InputSameDT=on
  Constant1 : Constant  Value=g_TargetStates.StateDetectedNotClassified*ones(g_MaxNumberTargets,1)
  No Alg Loop3 : UnitDelay  SampleTime=g_SampleTime
  New Target : Outport
  wires:
  Constant1/1 -> Check for new target/1
  Check for new target1/1 -> And 1/2
  No Alg Loop3/1 -> Check for new target1/2
  And 3/1 -> New Target/1
  And 1/1 -> And 3/1
  TargetStatus/1 -> Check for new target/2, Check for new target1/1, No Alg Loop3/1
  Check for new target/1 -> And 1/1

== system cooperative/UAV1/EmbeddedFlightSoftware/TargetManager/Sensed Target  Information ==
  In1 : Inport
  Bus Creator : BusCreator  Inputs=1
  Bus Selector5 : BusSelector  OutputSignals=ExternalTruth.TargetState
  PreventLoopback : Gain  SaturateOnIntegerOverflow=on  OutDataTypeStr=Inherit: Same as input  ParamDataTypeStr=Inherit: Same as input
  Out1 : Outport
  wires:
  Bus Creator/1 -> Out1/1  "SensedTargetInformation"
  Bus Selector5/1 -> PreventLoopback/1  "<TargetState>"
  In1/1 -> Bus Selector5/1
  PreventLoopback/1 -> Bus Creator/1  "Targets"

== system cooperative/UAV1/EmbeddedFlightSoftware/TargetManager/Target Status ==
  note: Target Status
      |
      | PURPOSE: This block is used to calculate and maintain the staus of each
      | of the targets. The block "Update Target Status" calls the
      | M-function "TargetStatus" to do the calculations.
      |
      |
      | IMPLEMENTATION:
      | - TargetStatusS - calls the MATLAB function "TargetStatus" to update the
      |      status of the targets.
      |
      | Target States:
      | 0 - Not Detected (~D)
      | 1 - Detected/Not Classified (D/~C)
      | 2 -  Classified/Not Attacked (C/~A)
      | 3 - Attacked/Not Killed (A/~K)
      | 4 - Killed/Not Verified (K/~V)
      | 5 - Verified  (V)
  Local (Comm) : Inport  SampleTime=g_SampleTime
  Combined ATR : Inport  Port=2  SampleTime=g_SampleTime
  SimBusIn : Inport  Port=3  SampleTime=g_SampleTime
  ComBusIn : Inport  Port=4  SampleTime=g_SampleTime
  Enable : EnablePort
  Bus Selector : BusSelector  OutputSignals=VehicleID,Time,EFS(com).RouteManager(com).TaskStatus.Last Task Finished,EFS(com).SensorManager(com).ATR Combined.NumberValidHeadings  OutputAsBus=on
  Bus Selector1 : BusSelector  OutputSignals=TargetStatus,TargetAttacked  OutputAsBus=on
  Bus Selector4 : BusSelector  OutputSignals=ExternalTruth.VehicleIsDead  OutputAsBus=on
  Demux : Demux  Outputs=[g_MaxNumberTargets 1]
  Mux2 : Mux  Inputs=3
  TargetStatusS : S-Function  FunctionName=TargetStatusS  Parameters=g_MaxNumberTargets,g_MaxNumberVehicles  EnableBusSupport=off
  "Write Last Combined ATR/BDA " : DataStoreWrite  DataStoreName=LastCombinedATR  SampleTime=g_SampleTime
  Write Last Vehicle Finished : DataStoreWrite  DataStoreName=LastVehicleFinished  SampleTime=g_SampleTime
  Target Status : Outport
  Changed Status : Outport  Port=2
  wires:
  Demux/2 -> Changed Status/1  "TargetStatus02"
  SimBusIn/1 -> Bus Selector4/1
  Bus Selector4/1 -> Write Last Vehicle Finished/1
  TargetStatusS/1 -> Demux/1  "TargetStatus"
  Demux/1 -> Target Status/1  "TargetStatus"
  Combined ATR/1 -> Mux2/2, "Write Last Combined ATR/BDA "/1
  ComBusIn/1 -> Bus Selector1/1
  Bus Selector/1 -> Mux2/1
  Bus Selector1/1 -> Mux2/3
  Local (Comm)/1 -> Bus Selector/1
  Mux2/1 -> TargetStatusS/1  "Target Manager"
